simulink model "pid_test"  (R2017b)
settings: Solver=ode3  StartTime=0.0  StopTime=10  FixedStep=0.001  RelTol=1e-3
libraries: simulink x1
settings Model: Creator=Administrator  LastModifiedBy=Administrator
settings OptimizationCC: DefaultParameterBehavior=Inlined  PassReuseOutputArgsAs=Individual arguments
settings DebuggingCC: ParameterTunabilityLossMsg=error
settings SFSimCC: MATLABDynamicMemAlloc=off
settings RTWCC: SystemTargetFile=ert.tlc  GenCodeOnly=on  TemplateMakefile=ert_default_tmf  GenerateReport=on  IncludeHyperlinkInReport=on  LaunchReport=on  GenerateTraceInfo=on  GenerateTraceReport=on  GenerateTraceReportSl=on  GenerateTraceReportSf=on  GenerateTraceReportEml=on
settings CodeAppCC: ForceParamTrailComments=on  IgnoreCustomStorageClasses=off  OperatorAnnotations=on  SimulinkDataObjDesc=on  SFDataObjDesc=on  InsertBlockDesc=on
settings ERTTargetCC: TargetLangStandard=C99 (ISO)  SupportContinuousTime=on  InlinedParameterPlacement=NonHierarchical  ERTCustomFileTemplate=example_file_process.tlc

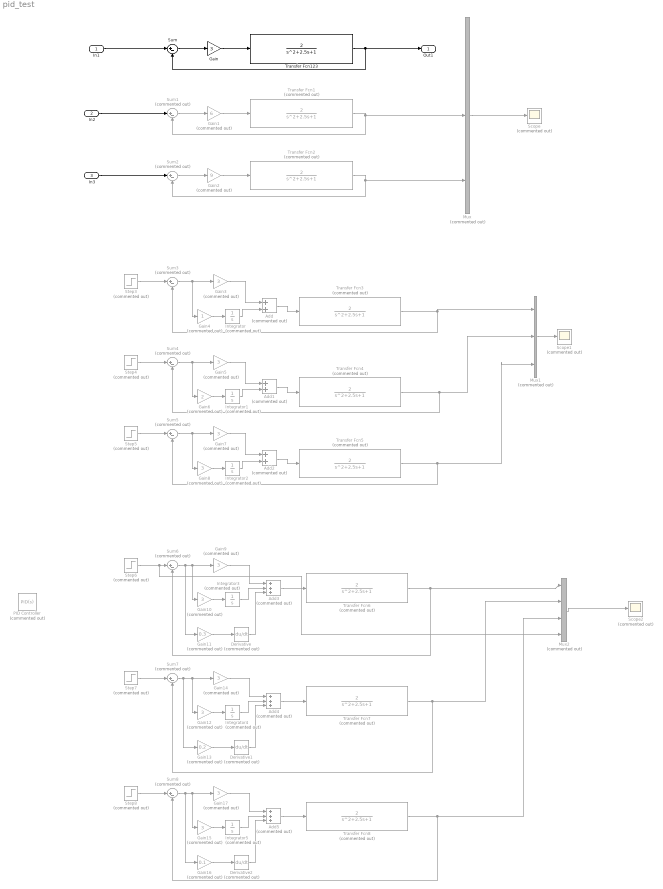
== system pid_test ==
  In1 : Inport
  In2 : Inport  Port=2
  In3 : Inport  Port=3
  Add : Sum  Commented=on
  Add1 : Sum  Commented=on
  Add2 : Sum  Commented=on
  Add3 : Sum  Commented=on  Inputs=+++
  Add4 : Sum  Commented=on  Inputs=+++
  Add5 : Sum  Commented=on  Inputs=+++
  Derivative : Derivative  Commented=on
  Derivative1 : Derivative  Commented=on
  Derivative2 : Derivative  Commented=on
  Gain : Gain  Gain=3
  Gain1 : Gain  Commented=on  Gain=6
  Gain{3,5,7..10,12,14..15,17} (10 alike) : Gain  Commented=on  Gain=3
  Gain11 : Gain  Commented=on  Gain=0.3
  Gain13 : Gain  Commented=on  Gain=0.2
  Gain16 : Gain  Commented=on  Gain=0.1
  Gain2 : Gain  Commented=on  Gain=9
  Gain4 : Gain  Commented=on
  Gain6 : Gain  Commented=on  Gain=2
  Integrator{,1..5} (6 alike) : Integrator  Commented=on
  Mux : Mux  Commented=on  Inputs=3
  Mux1 : Mux  Commented=on  Inputs=3
  Mux2 : Mux  Commented=on
  PID Controller : simulink/Continuous/PID Controller  Commented=on  Controller=PID  TimeDomain=Continuous-time  SampleTime=-1  IntegratorMethod=Forward Euler  FilterMethod=Forward Euler  Form=Parallel  UseFilter=on  ControllerParametersSource=internal  P=1  I=1  D=0  N=100  InitialConditionSource=internal  InitialConditionForIntegrator=0  InitialConditionForFilter=0  ExternalReset=none  LimitOutput=off  UpperSaturationLimit=inf  LowerSaturationLimit=-inf  LinearizeAsGain=on  AntiWindupMode=none  Kb=1  TrackingMode=off  Kt=1  PParamMin=[]  PParamMax=[]  IParamMin=[]  IParamMax=[]  DParamMin=[]  DParamMax=[]  NParamMin=[]  NParamMax=[]  KbParamMin=[]  KbParamMax=[]  KtParamMin=[]  KtParamMax=[]  POutMin=[]  POutMax=[]  IOutMin=[]  IOutMax=[]  DOutMin=[]  DOutMax=[]  NOutMin=[]  NOutMax=[]  KbOutMin=[]  KbOutMax=[]  KtOutMin=[]  KtOutMax=[]  IntegratorOutMin=[]  IntegratorOutMax=[]  FilterOutMin=[]  FilterOutMax=[]  SumOutMin=[]  SumOutMax=[]  SumI1OutMin=[]  SumI1OutMax=[]  SumI2OutMin=[]  SumI2OutMax=[]  SumI3OutMin=[]  SumI3OutMax=[]  SumDOutMin=[]  SumDOutMax=[]  SaturationOutMin=[]  SaturationOutMax=[]  IntegratorContinuousStateAttributes=''  IntegratorStateMustResolveToSignalObject=off  IntegratorRTWStateStorageClass=Auto  FilterContinuousStateAttributes=''  FilterStateMustResolveToSignalObject=off  FilterRTWStateStorageClass=Auto  DifferentiatorICPrevScaledInput=0  DifferentiatorOutMin=[]  DifferentiatorOutMax=[]  InitialConditionSetting=State (most efficient)  FilterDiffOutCoefMin=[]  FilterDiffOutCoefMax=[]  SumDenOutMin=[]  SumDenOutMax=[]  SumNumOutMin=[]  SumNumOutMax=[]  ReciprocalOutMin=[]  ReciprocalOutMax=[]  DivideOutMin=[]  DivideOutMax=[]  TunerSelectOption=Transfer Function Based (PID Tuner App)
  Scope : Scope  Commented=on
  Scope1 : Scope  Commented=on
  Scope2 : Scope  Commented=on
  Step{3..8} (6 alike) : Step  Commented=on  SampleTime=0
  Sum : Sum  Inputs=|+-
  Sum{1..8} (8 alike) : Sum  Commented=on  Inputs=|+-
  Transfer Fcn{1..8} (8 alike) : TransferFcn  Commented=on  Numerator=[2]  Denominator=[1 2.5 1]
  "Transfer Fcn123 " : TransferFcn  Numerator=[2]  Denominator=[1 2.5 1]
  Out1 : Outport
  wires:
  Mux/1 -> Scope/1
  "Transfer Fcn123 "/1 -> Sum/2, Out1/1
  Gain/1 -> "Transfer Fcn123 "/1
  In1/1 -> Sum/1
  Sum/1 -> Gain/1
  In2/1 -> Sum1/1
  Gain1/1 -> Transfer Fcn1/1
  Sum1/1 -> Gain1/1
  Transfer Fcn1/1 -> Sum1/2, Mux/2
  In3/1 -> Sum2/1
  Gain2/1 -> Transfer Fcn2/1
  Sum2/1 -> Gain2/1
  Transfer Fcn2/1 -> Sum2/2, Mux/3
  Gain3/1 -> Add/1
  Step3/1 -> Sum3/1
  Transfer Fcn3/1 -> Sum3/2, Mux1/1
  Sum3/1 -> Gain4/1, Gain3/1
  Add/1 -> Transfer Fcn3/1
  Gain4/1 -> Integrator/1
  Integrator/1 -> Add/2
  Sum4/1 -> Gain6/1, Gain5/1
  Step4/1 -> Sum4/1
  Transfer Fcn4/1 -> Sum4/2, Mux1/2
  Gain6/1 -> Integrator1/1
  Gain5/1 -> Add1/1
  Integrator1/1 -> Add1/2
  Add1/1 -> Transfer Fcn4/1
  Sum5/1 -> Gain8/1, Gain7/1
  Step5/1 -> Sum5/1
  Transfer Fcn5/1 -> Sum5/2, Mux1/3
  Gain8/1 -> Integrator2/1
  Gain7/1 -> Add2/1
  Integrator2/1 -> Add2/2
  Add2/1 -> Transfer Fcn5/1
  Mux1/1 -> Scope1/1
  Sum6/1 -> Gain11/1, Gain10/1, Gain9/1
  Step6/1 -> Mux2/4, Sum6/1
  Transfer Fcn6/1 -> Sum6/2, Mux2/1
  Gain10/1 -> Integrator3/1
  Gain9/1 -> Add3/1
  Integrator3/1 -> Add3/2
  Add3/1 -> Transfer Fcn6/1
  Gain11/1 -> Derivative/1
  Derivative/1 -> Add3/3
  Step7/1 -> Sum7/1
  Sum7/1 -> Gain13/1, Gain12/1, Gain14/1
  Derivative1/1 -> Add4/3
  Integrator4/1 -> Add4/2
  Add4/1 -> Transfer Fcn7/1
  Gain14/1 -> Add4/1
  Transfer Fcn7/1 -> Sum7/2, Mux2/2
  Gain12/1 -> Integrator4/1
  Gain13/1 -> Derivative1/1
  Step8/1 -> Sum8/1
  Sum8/1 -> Gain16/1, Gain15/1, Gain17/1
  Derivative2/1 -> Add5/3
  Integrator5/1 -> Add5/2
  Add5/1 -> Transfer Fcn8/1
  Gain17/1 -> Add5/1
  Transfer Fcn8/1 -> Sum8/2, Mux2/3
  Gain15/1 -> Integrator5/1
  Gain16/1 -> Derivative2/1
  Mux2/1 -> Scope2/1
